simulink model "Q2"  (R2023a)
settings: Solver=FixedStepAuto  StartTime=0.0  StopTime=20  FixedStep=0.0001  RelTol=1e-3
settings Model: Creator=DELL  LastModifiedBy=DELL

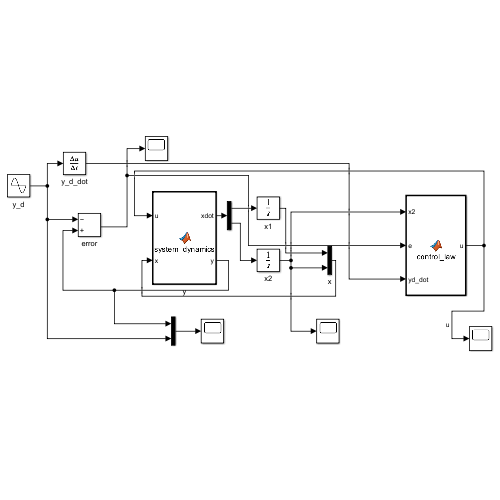
[thumbnail: Simulink's stored preview of the top-level diagram]
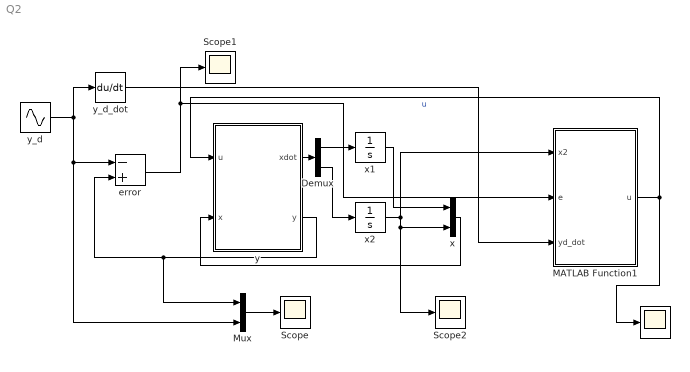
== system Q2 ==
  " " : Scope
  Demux : Demux  Outputs=2
  MATLAB Function1 : MATLAB Function  TreatAsAtomicUnit=on
  Mux : Mux  Inputs=2
  Scope : Scope
  Scope1 : Scope
  Scope2 : Scope
  error : Sum  Inputs=-+
  x : Mux  Inputs=2
  x1 : Integrator
  x2 : Integrator
  y : MATLAB Function  TreatAsAtomicUnit=on
  y_d : Sin  SampleTime=0
  y_d_dot : Derivative
  wires:
  y_d/1 -> Mux/2, error/1, y_d_dot/1
  error/1 -> Scope1/1, MATLAB Function1/2(e)
  y_d_dot/1 -> MATLAB Function1/3(yd_dot)
  MATLAB Function1/1(u) -> " "/1, y/1(u)  "u"
  Mux/1 -> Scope/1
  x1/1 -> x/1
  x/1 -> y/2(x)
  x2/1 -> Scope2/1, x/2, MATLAB Function1/1(x2)
  y/1(xdot) -> Demux/1
  Demux/1 -> x1/1
  Demux/2 -> x2/1
  y/2(y) -> Mux/1, error/2

== matlab function Q2/MATLAB Function1 ==
  data: u output; x2 input; e input; yd_dot input
function u = control_law(x2, e, yd_dot)
    u = -x2^3 - e + yd_dot;
end

== matlab function Q2/y ==
  data: xdot output; u input; y output; x input
function [xdot, y] = system_dynamics(u, x)
    % Validate input dimensions
    coder.extrinsic('error');
    if ~isequal(size(x), [2, 1])
        error('Input x must be a 2x1 vector');
    end
    if ~isscalar(u)
        error('Input u must be a scalar');
    end

    % System dynamics
    x1 = x(1);
    x2 = x(2);
    xdot = [x2^3 + u; u];
    y = x1;

    % Ensure output dimensions
    xdot = reshape(xdot, [2, 1]);
    y = reshape(y, [1, 1]);
end
